simulink model "vehicle_cornering_aero_model"  (R2025b)
settings: Solver=VariableStepAuto  StartTime=0.0  StopTime=100  RelTol=1e-3
model workspace (MAT data in the model file):
  xdot_o : Simulink.Parameter (value not decoded)
undefined symbols (not defined in the file or in its folder): Ab, Af, brakeBias, cf, Cl, cr, Gamma, gearRatio, hg, Ixx, Kpf, Kpr, l, m, maxPower, maxRev, maxWhlAng, Prs, RCf, RCr, rho, SteerFrq, tireD, track, vref, wd
libraries: simulink_extras x4, simulink x3, vehdynlibtirecommon x3, sharedtransform x3, autolibutils x2, vehdynlibdriver x1, vehdynlibtire x1, autolibshared x1
(part 2 of 2)

== matlab function vehicle_cornering_aero_model/ロール剛性/ロールモーメント計算 ==
  data: ay input; Mroll output; m parameter; RCf parameter; RCr parameter; wd parameter; hg parameter
function Mroll = fcn(ay, m, RCf, RCr, wd, hg)

%ロール軸からの重心高高さ
RCm = RCf + ((wd-0)/(1-0))*(RCr-RCf);

%ロールモーメント計算
Mroll = m*ay*9.806*(hg-RCm);

== matlab function vehicle_cornering_aero_model/ロール剛性/ロール方向運動方程式 ==
  data: phidot input; phidotdot output; phi input; Mroll input; Kpf parameter; Kpr parameter; cf parameter; cr parameter; track parameter; Ixx parameter
function phidotdot = fcn(phidot, phi, Mroll, Kpf, Kpr, cf, cr, track, Ixx)

TF = track(1,1);
TR = track(1,2);
%総ロール剛性計算
kp = Kpf + Kpr;

%ロール減衰係数計算
cpf = 2*cf*(TF/2)^2;
cpr = 2*cr*(TR/2)^2;

%総ロール減衰計算
cp = cpf+cpr;

%ロ―ル方向の運動方程式
phidotdot = (Mroll-cp*phidot-kp*phi)/Ixx;
